simulink model "k1visetmyp"  (Simulink 8.6)
settings: Solver=ode45  StartTime=0.0  StopTime=10.0  RelTol=1e-3
libraries: cdsIPCx x50, cdsFilt x11, cdsCDI64 x6, cdsCDO64 x6, BIO_CD_DECODE_MASTER x6, BIO_CD_ENCODE_MASTER x5, CHK_DIO x5, dac x3, cdsBit2Word x2, cdsAdcx0 x1, cdsAdcx1 x1, TYPEA_MASTER x1
(part 1 of 2)
settings Model: Creator=controls  LastModifiedBy=controls
settings DataIOCC: SignalLoggingSaveFormat=Dataset
settings OptimizationCC: ExpressionDepthLimit=128
settings DebuggingCC: UnderspecifiedInitializationDetection=Simplified  MergeDetectMultiDrivingBlocksExec=error  SolverPrmCheckMsg=none  FcnCallInpInsideContextMsg=EnableAllAsError  StateNameClashWarn=none
settings GRTTargetCC: CombineOutputUpdateFcns=on  GRTInterface=off

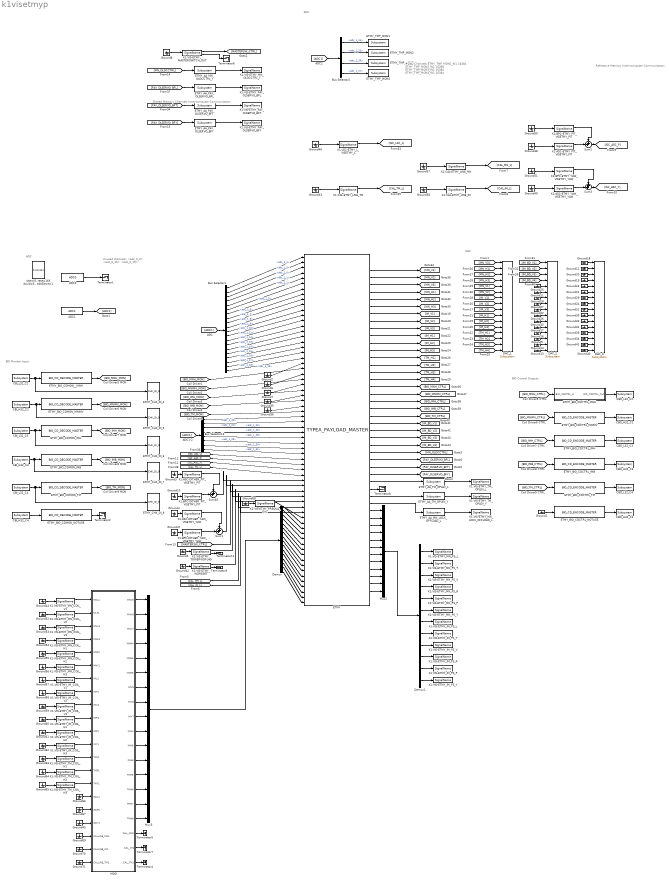
== system k1visetmyp ==
  note: BIO Monitor Input
  note: BIO Control Outputs
  note: DAC
  note: ADC
  note: Refrective Memory
      | Inner-computer Communication
  note: Unused channels:
      | <adc_0_3>
      | <adc_0_15>
      | <adc_0_19>
  note: Shared Memory Channels
      | Inner-computer Communication
  note: #DAQ Channels
      | ETMY_TMP_MON1_IN1 16384
      | ETMY_TMP_MON2_IN1 16384
      | ETMY_TMP_MON3_IN1 16384
      | ETMY_TMP_MON4_IN1 16384
  note: ADC
  ADC0 : cdsAdcx0/ADC0  Tag=cdsAdc  Description=|
      | type-GSC_16AI64SSA
      | card_num=0
      settings: AttributesFormatString=%<Description>\n%<Tag>
  ADC1 : cdsAdcx1/ADC1  Tag=cdsAdc  Description=|
      | type-GSC_16AI64SSA
      | card_num=1
      settings: AttributesFormatString=%<Description>\n%<Tag>
  Bus Selector1 : BusSelector  OutputSignals=adc_1_4,adc_1_5,adc_1_0,adc_1_1,adc_1_2,adc_1_3,adc_1_6,adc_1_7,adc_1_8,adc_1_9,adc_1_10,adc_1_11,adc_1_12,adc_1_13,adc_1_14,adc_1_15,adc_1_16,adc_1_17,adc_1_18,adc_1_19
  Bus Selector13 : BusSelector  OutputSignals=adc_1_20,adc_1_21,adc_1_22,adc_1_23,adc_1_28,adc_1_29,adc_1_30,adc_1_31
  Bus Selector2 : BusSelector  OutputSignals=adc_1_24,adc_1_25,adc_1_26,adc_1_27
  CBI_H32_C2 : cdsCDI64/Subsystem  Tag=cdsCDI64  Description=card_num=5
      settings: AttributesFormatString=%<Tag>\n%<Description>
  CBI_H32_C3 : cdsCDI64/Subsystem  Tag=cdsCDI64  Description=card_num=7
      settings: AttributesFormatString=%<Tag>\n%<Description>
  CBI_H32_C4 : cdsCDI64/Subsystem  Tag=cdsCDI64  Description=card_num=9
      settings: AttributesFormatString=%<Tag>\n%<Description>
  CBI_L32_C2 : cdsCDI64/Subsystem  Tag=cdsCDI64  Description=card_num=4
      settings: AttributesFormatString=%<Tag>\n%<Description>
  CBI_L32_C3 : cdsCDI64/Subsystem  Tag=cdsCDI64  Description=card_num=6
      settings: AttributesFormatString=%<Tag>\n%<Description>
  CBI_L32_C4 : cdsCDI64/Subsystem  Tag=cdsCDI64  Description=card_num=8
      settings: AttributesFormatString=%<Tag>\n%<Description>
  CBO_H32_C2 : cdsCDO64/Subsystem  Tag=cdsCDO64  Description=card_num=5
      settings: AttributesFormatString=%<Tag>\n%<Description>
  CBO_H32_C3 : cdsCDO64/Subsystem  Tag=cdsCDO64  Description=card_num=7
      settings: AttributesFormatString=%<Tag>\n%<Description>
  CBO_H32_C4 : cdsCDO64/Subsystem  Tag=cdsCDO64  Description=card_num=9
      settings: AttributesFormatString=%<Tag>\n%<Description>
  CBO_L32_C2 : cdsCDO64/Subsystem  Tag=cdsCDO64  Description=card_num=4
      settings: AttributesFormatString=%<Tag>\n%<Description>
  CBO_L32_C3 : cdsCDO64/Subsystem  Tag=cdsCDO64  Description=card_num=6
      settings: AttributesFormatString=%<Tag>\n%<Description>
  CBO_L32_C4 : cdsCDO64/Subsystem  Tag=cdsCDO64  Description=card_num=8
      settings: AttributesFormatString=%<Tag>\n%<Description>
  DAC_0 : dac/Subsystem  Description=|
      | type=GSC_16AO16,
      | card_num=0
      settings: AttributesFormatString=%<Description>
  DAC_1 : dac/Subsystem  Description=|
      | type=GSC_16AO16,
      | card_num=1
      settings: AttributesFormatString=%<Description>
  DAC_2 : dac/Subsystem  Description=|
      | type=GSC_16AO16,
      | card_num=2
      settings: AttributesFormatString=%<Description>
  Demux : Demux  Outputs=16
  Demux1 : Demux  Outputs=12
  ETMY : TYPEA_MASTER/TYPEA_PAYLOAD_MASTER
  ETMY_AA_MN_LOCK_OFFLOAD_L : cdsFilt/Subsystem  Tag=cdsFilt  Description=|
      | Purpose:                                                                                                                                                                                                                                  
      | Standard CDS IIR filter module.                                                                                                                                                                                                           
      |                                                                                                                                                                                                                                           
      | Operation:                                                                                                                                                                                                                                
      | Consists of 10 second order section IIR filters, plus a ramped gain stage. In FE code, also provides pre-defined test points and excitation channel inputs. The filter coefficients are defined in the LIGO system using the 'foton' tool.
      |                                                                                                                                                                                                                                           
      | Usage:                                                                                                                                                                                                                                    
      | Name the part with the desired filter module name.
      settings: AttributesFormatString=%<Tag>
  ETMY_AA_MN_OLDCCTRL_Y : cdsFilt/Subsystem  Tag=cdsFilt  Description=|
      | Purpose:                                                                                                                                                                                                                                  
      | Standard CDS IIR filter module.                                                                                                                                                                                                           
      |                                                                                                                                                                                                                                           
      | Operation:                                                                                                                                                                                                                                
      | Consists of 10 second order section IIR filters, plus a ramped gain stage. In FE code, also provides pre-defined test points and excitation channel inputs. The filter coefficients are defined in the LIGO system using the 'foton' tool.
      |                                                                                                                                                                                                                                           
      | Usage:                                                                                                                                                                                                                                    
      | Name the part with the desired filter module name.
      settings: AttributesFormatString=%<Tag>
  ETMY_AA_PAY_OLSERVO_BFL : cdsFilt/Subsystem  Tag=cdsFilt  Description=|
      | Purpose:                                                                                                                                                                                                                                  
      | Standard CDS IIR filter module.                                                                                                                                                                                                           
      |                                                                                                                                                                                                                                           
      | Operation:                                                                                                                                                                                                                                
      | Consists of 10 second order section IIR filters, plus a ramped gain stage. In FE code, also provides pre-defined test points and excitation channel inputs. The filter coefficients are defined in the LIGO system using the 'foton' tool.
      |                                                                                                                                                                                                                                           
      | Usage:                                                                                                                                                                                                                                    
      | Name the part with the desired filter module name.
      settings: AttributesFormatString=%<Tag>
  ETMY_AA_PAY_OLSERVO_BFT : cdsFilt/Subsystem  Tag=cdsFilt  Description=|
      | Purpose:                                                                                                                                                                                                                                  
      | Standard CDS IIR filter module.                                                                                                                                                                                                           
      |                                                                                                                                                                                                                                           
      | Operation:                                                                                                                                                                                                                                
      | Consists of 10 second order section IIR filters, plus a ramped gain stage. In FE code, also provides pre-defined test points and excitation channel inputs. The filter coefficients are defined in the LIGO system using the 'foton' tool.
      |                                                                                                                                                                                                                                           
      | Usage:                                                                                                                                                                                                                                    
      | Name the part with the desired filter module name.
      settings: AttributesFormatString=%<Tag>
  ETMY_AA_PAY_OLSERVO_BFY : cdsFilt/Subsystem  Tag=cdsFilt  Description=|
      | Purpose:                                                                                                                                                                                                                                  
      | Standard CDS IIR filter module.                                                                                                                                                                                                           
      |                                                                                                                                                                                                                                           
      | Operation:                                                                                                                                                                                                                                
      | Consists of 10 second order section IIR filters, plus a ramped gain stage. In FE code, also provides pre-defined test points and excitation channel inputs. The filter coefficients are defined in the LIGO system using the 'foton' tool.
      |                                                                                                                                                                                                                                           
      | Usage:                                                                                                                                                                                                                                    
      | Name the part with the desired filter module name.
      settings: AttributesFormatString=%<Tag>
  ETMY_AA_TM_OPLEV_L : cdsFilt/Subsystem  Tag=cdsFilt  Description=|
      | Purpose:                                                                                                                                                                                                                                  
      | Standard CDS IIR filter module.                                                                                                                                                                                                           
      |                                                                                                                                                                                                                                           
      | Operation:                                                                                                                                                                                                                                
      | Consists of 10 second order section IIR filters, plus a ramped gain stage. In FE code, also provides pre-defined test points and excitation channel inputs. The filter coefficients are defined in the LIGO system using the 'foton' tool.
      |                                                                                                                                                                                                                                           
      | Usage:                                                                                                                                                                                                                                    
      | Name the part with the desired filter module name.
      settings: AttributesFormatString=%<Tag>
  ETMY_AA_TM_OPLEV_Y : cdsFilt/Subsystem  Tag=cdsFilt  Description=|
      | Purpose:                                                                                                                                                                                                                                  
      | Standard CDS IIR filter module.                                                                                                                                                                                                           
      |                                                                                                                                                                                                                                           
      | Operation:                                                                                                                                                                                                                                
      | Consists of 10 second order section IIR filters, plus a ramped gain stage. In FE code, also provides pre-defined test points and excitation channel inputs. The filter coefficients are defined in the LIGO system using the 'foton' tool.
      |                                                                                                                                                                                                                                           
      | Usage:                                                                                                                                                                                                                                    
      | Name the part with the desired filter module name.
      settings: AttributesFormatString=%<Tag>
  ETMY_BIO_CDCTRL_IMB : BIO_CD_ENCODE_MASTER/BIO_CD_ENCODE_MASTER
  ETMY_BIO_CDCTRL_IMH : BIO_CD_ENCODE_MASTER/BIO_CD_ENCODE_MASTER
  ETMY_BIO_CDCTRL_MNH : Subsystem
  ETMY_BIO_CDCTRL_MNIMV : BIO_CD_ENCODE_MASTER/BIO_CD_ENCODE_MASTER
  ETMY_BIO_CDCTRL_NOTUSE : BIO_CD_ENCODE_MASTER/BIO_CD_ENCODE_MASTER
  ETMY_BIO_CDCTRL_TM : BIO_CD_ENCODE_MASTER/BIO_CD_ENCODE_MASTER
  ETMY_BIO_CDMON_IMB : BIO_CD_DECODE_MASTER/BIO_CD_DECODE_MASTER
  ETMY_BIO_CDMON_IMH : BIO_CD_DECODE_MASTER/BIO_CD_DECODE_MASTER
  ETMY_BIO_CDMON_MNIMV : BIO_CD_DECODE_MASTER/BIO_CD_DECODE_MASTER
  ETMY_BIO_CDMON_NOTUSE : BIO_CD_DECODE_MASTER/BIO_CD_DECODE_MASTER
  ETMY_BIO_CDMON_TM : BIO_CD_DECODE_MASTER/BIO_CD_DECODE_MASTER
  ETMY_BIO_CDMON__MNH : BIO_CD_DECODE_MASTER/BIO_CD_DECODE_MASTER
  ETMY_CHK_DI_{4..8} (5 alike) : CHK_DIO/CHK_DI_0
  ETMY_TMP_MON1 : cdsFilt/Subsystem  Tag=cdsFilt  Description=|
      | Purpose:                                                                                                                                                                                                                                  
      | Standard CDS IIR filter module.                                                                                                                                                                                                           
      |                                                                                                                                                                                                                                           
      | Operation:                                                                                                                                                                                                                                
      | Consists of 10 second order section IIR filters, plus a ramped gain stage. In FE code, also provides pre-defined test points and excitation channel inputs. The filter coefficients are defined in the LIGO system using the 'foton' tool.
      |                                                                                                                                                                                                                                           
      | Usage:                                                                                                                                                                                                                                    
      | Name the part with the desired filter module name.
      settings: AttributesFormatString=%<Tag>
  ETMY_TMP_MON2 : cdsFilt/Subsystem  Tag=cdsFilt  Description=|
      | Purpose:                                                                                                                                                                                                                                  
      | Standard CDS IIR filter module.                                                                                                                                                                                                           
      |                                                                                                                                                                                                                                           
      | Operation:                                                                                                                                                                                                                                
      | Consists of 10 second order section IIR filters, plus a ramped gain stage. In FE code, also provides pre-defined test points and excitation channel inputs. The filter coefficients are defined in the LIGO system using the 'foton' tool.
      |                                                                                                                                                                                                                                           
      | Usage:                                                                                                                                                                                                                                    
      | Name the part with the desired filter module name.
      settings: AttributesFormatString=%<Tag>
  ETMY_TMP_MON3 : cdsFilt/Subsystem  Tag=cdsFilt  Description=|
      | Purpose:                                                                                                                                                                                                                                  
      | Standard CDS IIR filter module.                                                                                                                                                                                                           
      |                                                                                                                                                                                                                                           
      | Operation:                                                                                                                                                                                                                                
      | Consists of 10 second order section IIR filters, plus a ramped gain stage. In FE code, also provides pre-defined test points and excitation channel inputs. The filter coefficients are defined in the LIGO system using the 'foton' tool.
      |                                                                                                                                                                                                                                           
      | Usage:                                                                                                                                                                                                                                    
      | Name the part with the desired filter module name.
      settings: AttributesFormatString=%<Tag>
  ETMY_TMP_MON4 : cdsFilt/Subsystem  Tag=cdsFilt  Description=|
      | Purpose:                                                                                                                                                                                                                                  
      | Standard CDS IIR filter module.                                                                                                                                                                                                           
      |                                                                                                                                                                                                                                           
      | Operation:                                                                                                                                                                                                                                
      | Consists of 10 second order section IIR filters, plus a ramped gain stage. In FE code, also provides pre-defined test points and excitation channel inputs. The filter coefficients are defined in the LIGO system using the 'foton' tool.
      |                                                                                                                                                                                                                                           
      | Usage:                                                                                                                                                                                                                                    
      | Name the part with the desired filter module name.
      settings: AttributesFormatString=%<Tag>
  Ground{1..71} (71 alike) : Ground
  K1:ASC-DITHER_PIT_VISETMY_PIT : cdsIPCx/SignalName  Tag=cdsIPCx_RFM  Description=card=1
      settings: AttributesFormatString=%<Description>\n%<Tag>
  K1:ASC-DITHER_YAW_VISETMY_YAW : cdsIPCx/SignalName  Tag=cdsIPCx_RFM  Description=card=1
      settings: AttributesFormatString=%<Description>\n%<Tag>
  K1:ASC-ETMY_PIT_VISETMY_PIT : cdsIPCx/SignalName  Tag=cdsIPCx_RFM  Description=card=1
      settings: AttributesFormatString=%<Description>\n%<Tag>
  K1:ASC-ETMY_YAW_VISETMY_YAW : cdsIPCx/SignalName  Tag=cdsIPCx_RFM  Description=card=1
      settings: AttributesFormatString=%<Description>\n%<Tag>
  K1:BPC-DITHER_PIT_VISETMY_PIT : cdsIPCx/SignalName  Tag=cdsIPCx_RFM  Description=card=1
      settings: AttributesFormatString=%<Description>\n%<Tag>
  K1:BPC-DITHER_YAW_VISETMY_YAW : cdsIPCx/SignalName  Tag=cdsIPCx_RFM  Description=card=1
      settings: AttributesFormatString=%<Description>\n%<Tag>
  K1:BPC-ETMY_PIT_VISETMY_PIT : cdsIPCx/SignalName  Tag=cdsIPCx_RFM  Description=card=1
      settings: AttributesFormatString=%<Description>\n%<Tag>
  K1:BPC-ETMY_YAW_VISETMY_YAW : cdsIPCx/SignalName  Tag=cdsIPCx_RFM  Description=card=1
      settings: AttributesFormatString=%<Description>\n%<Tag>
  K1:CAL-ETMY_LINE_IM : cdsIPCx/SignalName  Tag=cdsIPCx_RFM  Description=card=1
      settings: AttributesFormatString=%<Description>\n%<Tag>
  K1:CAL-ETMY_LINE_MN : cdsIPCx/SignalName  Tag=cdsIPCx_RFM  Description=card=1
      settings: AttributesFormatString=%<Description>\n%<Tag>
  K1:CAL-ETMY_LINE_TM : cdsIPCx/SignalName  Tag=cdsIPCx_RFM  Description=card=1
      settings: AttributesFormatString=%<Description>\n%<Tag>
  K1:LSC-ETMY_L_VISETMY_L : cdsIPCx/SignalName  Tag=cdsIPCx_RFM  Description=card=1
      settings: AttributesFormatString=%<Description>\n%<Tag>
  K1:VIS-ETMY_IM_COIL_H1 : cdsIPCx/SignalName  Tag=cdsIPCx_SHMEM  Description=Inter-Process Communication via Shared memory.
      settings: AttributesFormatString=%<Tag>
  K1:VIS-ETMY_IM_COIL_H2 : cdsIPCx/SignalName  Tag=cdsIPCx_SHMEM  Description=Inter-Process Communication via Shared memory.
      settings: AttributesFormatString=%<Tag>
  K1:VIS-ETMY_IM_COIL_H3 : cdsIPCx/SignalName  Tag=cdsIPCx_SHMEM  Description=Inter-Process Communication via Shared memory.
      settings: AttributesFormatString=%<Tag>
  K1:VIS-ETMY_IM_COIL_V1 : cdsIPCx/SignalName  Tag=cdsIPCx_SHMEM  Description=Inter-Process Communication via Shared memory.
      settings: AttributesFormatString=%<Tag>
  K1:VIS-ETMY_IM_COIL_V2 : cdsIPCx/SignalName  Tag=cdsIPCx_SHMEM  Description=Inter-Process Communication via Shared memory.
      settings: AttributesFormatString=%<Tag>
  K1:VIS-ETMY_IM_COIL_V3 : cdsIPCx/SignalName  Tag=cdsIPCx_SHMEM  Description=Inter-Process Communication via Shared memory.
      settings: AttributesFormatString=%<Tag>
  K1:VIS-ETMY_MN_COIL_H1 : cdsIPCx/SignalName  Tag=cdsIPCx_SHMEM  Description=Inter-Process Communication via Shared memory.
      settings: AttributesFormatString=%<Tag>
  K1:VIS-ETMY_MN_COIL_H2 : cdsIPCx/SignalName  Tag=cdsIPCx_SHMEM  Description=Inter-Process Communication via Shared memory.
      settings: AttributesFormatString=%<Tag>
  K1:VIS-ETMY_MN_COIL_H3 : cdsIPCx/SignalName  Tag=cdsIPCx_SHMEM  Description=Inter-Process Communication via Shared memory.
      settings: AttributesFormatString=%<Tag>
  K1:VIS-ETMY_MN_COIL_V1 : cdsIPCx/SignalName  Tag=cdsIPCx_SHMEM  Description=Inter-Process Communication via Shared memory.
      settings: AttributesFormatString=%<Tag>
  K1:VIS-ETMY_MN_COIL_V2 : cdsIPCx/SignalName  Tag=cdsIPCx_SHMEM  Description=Inter-Process Communication via Shared memory.
      settings: AttributesFormatString=%<Tag>
  K1:VIS-ETMY_MN_COIL_V3 : cdsIPCx/SignalName  Tag=cdsIPCx_SHMEM  Description=Inter-Process Communication via Shared memory.
      settings: AttributesFormatString=%<Tag>
  K1:VIS-ETMY_TM_COIL_H1 : cdsIPCx/SignalName  Tag=cdsIPCx_SHMEM  Description=Inter-Process Communication via Shared memory.
      settings: AttributesFormatString=%<Tag>
  K1:VIS-ETMY_TM_COIL_H2 : cdsIPCx/SignalName  Tag=cdsIPCx_SHMEM  Description=Inter-Process Communication via Shared memory.
      settings: AttributesFormatString=%<Tag>
  K1:VIS-ETMY_TM_COIL_H3 : cdsIPCx/SignalName  Tag=cdsIPCx_SHMEM  Description=Inter-Process Communication via Shared memory.
      settings: AttributesFormatString=%<Tag>
  K1:VIS-ETMY_IM_PS_L : cdsIPCx/SignalName  Tag=cdsIPCx_SHMEM  Description=Inter-Process Communication via Shared memory.
      settings: AttributesFormatString=%<Tag>
  K1:VIS-ETMY_IM_PS_P : cdsIPCx/SignalName  Tag=cdsIPCx_SHMEM  Description=Inter-Process Communication via Shared memory.
      settings: AttributesFormatString=%<Tag>
  K1:VIS-ETMY_IM_PS_R : cdsIPCx/SignalName  Tag=cdsIPCx_SHMEM  Description=Inter-Process Communication via Shared memory.
      settings: AttributesFormatString=%<Tag>
  K1:VIS-ETMY_IM_PS_T : cdsIPCx/SignalName  Tag=cdsIPCx_SHMEM  Description=Inter-Process Communication via Shared memory.
      settings: AttributesFormatString=%<Tag>
  K1:VIS-ETMY_IM_PS_V : cdsIPCx/SignalName  Tag=cdsIPCx_SHMEM  Description=Inter-Process Communication via Shared memory.
      settings: AttributesFormatString=%<Tag>
  K1:VIS-ETMY_IM_PS_Y : cdsIPCx/SignalName  Tag=cdsIPCx_SHMEM  Description=Inter-Process Communication via Shared memory.
      settings: AttributesFormatString=%<Tag>
  K1:VIS-ETMY_MASTERSWITCH_OUT : cdsIPCx/SignalName  Tag=cdsIPCx_SHMEM  Description=Inter-Process Communication via Shared memory.
      settings: AttributesFormatString=%<Tag>
  K1:VIS-ETMY_MN_LOCK_OFFLOAD_L : cdsIPCx/SignalName  Tag=cdsIPCx_SHMEM  Description=Inter-Process Communication via Shared memory.
      settings: AttributesFormatString=%<Tag>
  K1:VIS-ETMY_MN_OLDCCTRL_Y : cdsIPCx/SignalName  Tag=cdsIPCx_SHMEM  Description=Inter-Process Communication via Shared memory.
      settings: AttributesFormatString=%<Tag>
  K1:VIS-ETMY_MN_PS_L : cdsIPCx/SignalName  Tag=cdsIPCx_SHMEM  Description=Inter-Process Communication via Shared memory.
      settings: AttributesFormatString=%<Tag>
  K1:VIS-ETMY_MN_PS_P : cdsIPCx/SignalName  Tag=cdsIPCx_SHMEM  Description=Inter-Process Communication via Shared memory.
      settings: AttributesFormatString=%<Tag>
  K1:VIS-ETMY_MN_PS_R : cdsIPCx/SignalName  Tag=cdsIPCx_SHMEM  Description=Inter-Process Communication via Shared memory.
      settings: AttributesFormatString=%<Tag>
  K1:VIS-ETMY_MN_PS_T : cdsIPCx/SignalName  Tag=cdsIPCx_SHMEM  Description=Inter-Process Communication via Shared memory.
      settings: AttributesFormatString=%<Tag>
  K1:VIS-ETMY_MN_PS_V : cdsIPCx/SignalName  Tag=cdsIPCx_SHMEM  Description=Inter-Process Communication via Shared memory.
      settings: AttributesFormatString=%<Tag>
  K1:VIS-ETMY_MN_PS_Y : cdsIPCx/SignalName  Tag=cdsIPCx_SHMEM  Description=Inter-Process Communication via Shared memory.
      settings: AttributesFormatString=%<Tag>
  K1:VIS-ETMY_PAY_OLSERVO_BFL : cdsIPCx/SignalName  Tag=cdsIPCx_SHMEM  Description=Inter-Process Communication via Shared memory.
      settings: AttributesFormatString=%<Tag>
  K1:VIS-ETMY_PAY_OLSERVO_BFT : cdsIPCx/SignalName  Tag=cdsIPCx_SHMEM  Description=Inter-Process Communication via Shared memory.
      settings: AttributesFormatString=%<Tag>
  K1:VIS-ETMY_PAY_OLSERVO_BFY : cdsIPCx/SignalName  Tag=cdsIPCx_SHMEM  Description=Inter-Process Communication via Shared memory.
      settings: AttributesFormatString=%<Tag>
  K1:VIS-ETMY_PREQUA_EXC : cdsIPCx/SignalName  Tag=cdsIPCx_SHMEM  Description=Inter-Process Communication via Shared memory.
      settings: AttributesFormatString=%<Tag>
  K1:VIS-ETMY_TM_OPLEV_L : cdsIPCx/SignalName  Tag=cdsIPCx_SHMEM  Description=Inter-Process Communication via Shared memory.
      settings: AttributesFormatString=%<Tag>
  K1:VIS-ETMY_TM_OPLEV_Y : cdsIPCx/SignalName  Tag=cdsIPCx_SHMEM  Description=Inter-Process Communication via Shared memory.
      settings: AttributesFormatString=%<Tag>
  K1:VIS-ETMY_TOWERWDFLAG : cdsIPCx/SignalName  Tag=cdsIPCx_SHMEM  Description=Inter-Process Communication via Shared memory.
      settings: AttributesFormatString=%<Tag>
  K1:VIS-ETMY_WDRESET : cdsIPCx/SignalName  Tag=cdsIPCx_SHMEM  Description=Inter-Process Communication via Shared memory.
      settings: AttributesFormatString=%<Tag>
  MOD : Subsystem  Tag=top_names
  Mux2 : Mux  Inputs=12
  Mux3 : Mux  Inputs=16
  Sum{1..3,45} (4 alike) : Sum  Inputs=++|
  Terminator{1..8,12} (9 alike) : Terminator
  site=K1 rate=16K dcuid=64 host=k1ey1 specific_cpu=3 adcSlave=1 : cdsParameters/Subsystem  Tag=cdsParameters  Description=|
      | Purpose:                                                                                                                                                                                                                                
      | Provide system parameters to the FE code generator to properly configure the generated EPICS names, rep rate of the FE controller, and the Data Acquisition node ID for proper storage of data from this FE controller.                 
      |                                                                                                                                                                                                                                         
      | Useage:                                                                                                                                                                                                                                 
      | The part NAME field is used to identify the FE parameters. It must be of the form:                                                                                                                                                      
      | site=                                                                                                                                                                                                                                   
      | rate=                                                                                                                                                                                                                                   
      | dcuid=                                                                                                                                                                                                                                  
      |                                                                                                                                                                                                                                         
      | Where:                                                                                                                                                                                                                                  
      | site= argument may be H1, H2, L1, M1, G1, either as a single argument or multiple, for example site=H1,H2. These are the only names allowed. These will become the first two characters of all EPICS and signal names (for example G1:).
      |                                                                                                                                                                                                                                         
      | rate= may be 2K, 16K, 32K, or 64K                                                                                                                                                                                                       
      |                                                                                                                                                                                                                                         
      | dcuid= is site specific ie it must be unique at each site.
      settings: AttributesFormatString=%<Tag>
  wires:
  ADC1/1 -> [ADC1]
  ETMY/1 -> [MN_V1]
  ETMY/2 -> [MN_V2]
  ETMY/3 -> [MN_V3]
  ETMY/4 -> [MN_H1]
  ETMY/6 -> [MN_H3]
  ETMY/7 -> [IM_V1]
  ETMY/8 -> [IM_V2]
  ETMY/9 -> [IM_V3]
  ETMY/11 -> [IM_H2]
  ETMY/12 -> [IM_H3]
  ETMY/13 -> [TM_H1]
  ETMY/14 -> [TM_H2]
  ETMY/16 -> [TM_H4]
  ETMY/17 -> [BIO_MNH_CTRL]
  ETMY/19 -> [BIO_IMH_CTRL]
  ETMY/18 -> [BIO_MNIMV_CTRL]
  ETMY/20 -> [BIO_IMB_CTRL]
  ETMY/21 -> [BIO_TM_CTRL]
  [ADC1] -> Bus Selector13/1
  [MN_V3] -> DAC_1/1
  [MN_H1] -> DAC_1/2
  [MN_H2] -> DAC_1/3
  [MN_H3] -> DAC_1/4
  [MN_V1] -> DAC_1/5
  [MN_V2] -> DAC_1/6
  [IM_V1] -> DAC_1/7
  [IM_V2] -> DAC_1/8
  [IM_V3] -> DAC_1/9
  [IM_H1] -> DAC_1/10
  [TM_H1] -> DAC_1/13
  [TM_H4] -> DAC_1/16
  [TM_H3] -> DAC_1/15
  [TM_H2] -> DAC_1/14
  [IM_H2] -> DAC_1/11
  [IM_H3] -> DAC_1/12
  [BIO_MNH_CTRL] -> ETMY_BIO_CDCTRL_MNH/1(BIO_CDCTRL_In)
  ETMY_BIO_CDCTRL_MNH/1(DIO_CDCTRL_Out) -> CBO_L32_C2/1
  [BIO_MNIMV_CTRL] -> ETMY_BIO_CDCTRL_MNIMV/1
  ETMY_BIO_CDCTRL_MNIMV/1 -> CBO_H32_C2/1
  [BIO_IMH_CTRL] -> ETMY_BIO_CDCTRL_IMH/1
  ETMY_BIO_CDCTRL_IMH/1 -> CBO_L32_C3/1
  [BIO_IMB_CTRL] -> ETMY_BIO_CDCTRL_IMB/1
  ETMY_BIO_CDCTRL_IMB/1 -> CBO_H32_C3/1
  [BIO_TM_CTRL] -> ETMY_BIO_CDCTRL_TM/1
  ETMY_BIO_CDCTRL_TM/1 -> CBO_L32_C4/1
  Ground1/1 -> ETMY_BIO_CDCTRL_NOTUSE/1
  ETMY_BIO_CDCTRL_NOTUSE/1 -> CBO_H32_C4/1
  CBI_L32_C2/1 -> ETMY_CHK_DI_4/1, ETMY_BIO_CDMON__MNH/1
  ETMY_BIO_CDMON__MNH/1 -> [BIO_MNH_MON]
  CBI_H32_C2/1 -> ETMY_CHK_DI_5/1, ETMY_BIO_CDMON_MNIMV/1
  ETMY_BIO_CDMON_MNIMV/1 -> [BIO_MNIMV_MON]
  CBI_L32_C3/1 -> ETMY_CHK_DI_6/1, ETMY_BIO_CDMON_IMH/1
  ETMY_BIO_CDMON_IMH/1 -> [BIO_IMH_MON]
  ETMY_BIO_CDMON_IMB/1 -> [BIO_IMB_MON]
  CBI_L32_C4/1 -> ETMY_CHK_DI_8/1, ETMY_BIO_CDMON_TM/1
  ETMY_BIO_CDMON_TM/1 -> [BIO_TM_MON]
  CBI_H32_C4/1 -> ETMY_BIO_CDMON_NOTUSE/1
  ETMY_BIO_CDMON_NOTUSE/1 -> Terminator2/1
  [IM_BD_V1] -> DAC_2/1
  [IM_BD_V2] -> DAC_2/2
  [IM_BD_V3] -> DAC_2/3
  [IM_BD_V4] -> DAC_2/4
  Ground25/1 -> DAC_2/5
  Ground11/1 -> DAC_2/6
  Ground28/1 -> DAC_2/7
  Ground27/1 -> DAC_2/8
  Ground22/1 -> DAC_2/9
  Ground26/1 -> DAC_2/10
  Ground15/1 -> DAC_2/11
  Ground17/1 -> DAC_2/12
  Ground16/1 -> DAC_2/13
  Ground9/1 -> DAC_2/14
  Ground14/1 -> DAC_2/15
  Ground13/1 -> DAC_2/16
  ETMY/22 -> [IM_BD_V1]
  ETMY/23 -> [IM_BD_V2]
  ETMY/24 -> [IM_BD_V3]
  ETMY/25 -> [IM_BD_V4]
  CBI_H32_C3/1 -> ETMY_CHK_DI_7/1, ETMY_BIO_CDMON_IMB/1
  ETMY/5 -> [MN_H2]
  ETMY/10 -> [IM_H1]
  ETMY/15 -> [TM_H3]
  [ADC1] -> Bus Selector1/1
  Bus Selector1/1 -> ETMY/1  "<adc_1_4>"
  Bus Selector1/2 -> ETMY/2  "<adc_1_5>"
  Bus Selector1/3 -> ETMY/3  "<adc_1_0>"
  Bus Selector1/4 -> ETMY/4  "<adc_1_1>"
  Bus Selector1/5 -> ETMY/5  "<adc_1_2>"
  Bus Selector1/6 -> ETMY/6  "<adc_1_3>"
  Bus Selector1/7 -> ETMY/7  "<adc_1_6>"
  Bus Selector1/8 -> ETMY/8  "<adc_1_7>"
  Bus Selector1/9 -> ETMY/9  "<adc_1_8>"
  Bus Selector1/10 -> ETMY/10  "<adc_1_9>"
  Bus Selector1/11 -> ETMY/11  "<adc_1_10>"
  Bus Selector1/12 -> ETMY/12  "<adc_1_11>"
  Bus Selector1/13 -> ETMY/13  "<adc_1_12>"
  Bus Selector1/14 -> ETMY/14  "<adc_1_13>"
  Bus Selector1/15 -> ETMY/15  "<adc_1_14>"
  Bus Selector1/16 -> ETMY/16  "<adc_1_15>"
  Bus Selector1/17 -> ETMY/17  "<adc_1_16>"
  Bus Selector1/18 -> ETMY/18  "<adc_1_17>"
  Bus Selector1/19 -> ETMY/19  "<adc_1_18>"
  Bus Selector1/20 -> ETMY/20  "<adc_1_19>"
  [BIO_MNH_MON] -> ETMY/22
  [BIO_MNIMV_MON] -> ETMY/24
  [BIO_IMH_MON] -> ETMY/26
  [BIO_IMB_MON] -> ETMY/28
  [BIO_TM_MON] -> ETMY/30
  Bus Selector13/2 -> ETMY/32  "<adc_1_21>"
  Bus Selector13/3 -> ETMY/33  "<adc_1_22>"
  Bus Selector13/4 -> ETMY/34  "<adc_1_23>"
  Bus Selector13/5 -> ETMY/35  "<adc_1_28>"
  Bus Selector13/6 -> ETMY/36  "<adc_1_29>"
  Bus Selector13/7 -> ETMY/37  "<adc_1_30>"
  Bus Selector13/8 -> ETMY/38  "<adc_1_31>"
  Bus Selector13/1 -> ETMY/31  "<adc_1_20>"
  [ISC_ASC_P] -> ETMY/40
  [ISC_ASC_Y] -> ETMY/41
  K1:VIS-ETMY_TOWERWDFLAG/2 -> Terminator12/1
  Ground5/1 -> K1:VIS-ETMY_TOWERWDFLAG/1
  ADC0/1 -> Terminator1/1
  Ground18/1 -> DAC_0/1
  Ground12/1 -> DAC_0/2
  Ground19/1 -> DAC_0/4
  Ground20/1 -> DAC_0/3
  Ground29/1 -> DAC_0/7
  Ground23/1 -> DAC_0/5
  Ground21/1 -> DAC_0/6
  Ground24/1 -> DAC_0/8
  Ground31/1 -> DAC_0/9
  Ground30/1 -> DAC_0/10
  Ground33/1 -> DAC_0/11
  Ground32/1 -> DAC_0/12
  Ground39/1 -> DAC_0/13
  Ground34/1 -> DAC_0/14
  Ground41/1 -> DAC_0/15
  Ground40/1 -> DAC_0/16
  K1:VIS-ETMY_WDRESET/2 -> Terminator3/1
  Ground42/1 -> K1:VIS-ETMY_WDRESET/1
  Ground46/1 -> K1:LSC-ETMY_L_VISETMY_L/1
  K1:LSC-ETMY_L_VISETMY_L/1 -> [ISC_LSC_L]
  K1:CAL-ETMY_LINE_TM/1 -> [CAL_TM_L]
  Ground43/1 -> K1:CAL-ETMY_LINE_TM/1
  [ISC_LSC_L] -> ETMY/39
  Ground2/1 -> ETMY/21
  Ground6/1 -> ETMY/23
  Ground7/1 -> ETMY/25
  Ground35/1 -> ETMY/27
  Ground36/1 -> ETMY/29
  K1:CAL-ETMY_LINE_MN/1 -> [CAL_MN_L]
  Ground37/1 -> K1:CAL-ETMY_LINE_MN/1
  K1:CAL-ETMY_LINE_IM/1 -> [CAL_IM_L]
  Ground38/1 -> K1:CAL-ETMY_LINE_IM/1
  K1:ASC-ETMY_PIT_VISETMY_PIT/1 -> Sum2/2
  K1:ASC-ETMY_YAW_VISETMY_YAW/1 -> Sum3/2
  Ground48/1 -> K1:ASC-ETMY_PIT_VISETMY_PIT/1
  Ground49/1 -> K1:ASC-ETMY_YAW_VISETMY_YAW/1
  Ground3/1 -> K1:ASC-DITHER_PIT_VISETMY_PIT/1
  Ground4/1 -> K1:ASC-DITHER_YAW_VISETMY_YAW/1
  ETMY_AA_MN_OLDCCTRL_Y/1 -> K1:VIS-ETMY_MN_OLDCCTRL_Y/1
  ETMY_AA_PAY_OLSERVO_BFY/1 -> K1:VIS-ETMY_PAY_OLSERVO_BFY/1
  ETMY_AA_PAY_OLSERVO_BFT/1 -> K1:VIS-ETMY_PAY_OLSERVO_BFT/1
  ETMY_AA_PAY_OLSERVO_BFL/1 -> K1:VIS-ETMY_PAY_OLSERVO_BFL/1
  [PAY_OLSERVO_BFY] -> ETMY_AA_PAY_OLSERVO_BFY/1
  [PAY_OLSERVO_BFT] -> ETMY_AA_PAY_OLSERVO_BFT/1
  [PAY_OLSERVO_BFL] -> ETMY_AA_PAY_OLSERVO_BFL/1
  [MN_OLDCCTRL] -> ETMY_AA_MN_OLDCCTRL_Y/1
  ETMY_AA_TM_OPLEV_L/1 -> K1:VIS-ETMY_TM_OPLEV_L/1
  ETMY_AA_TM_OPLEV_Y/1 -> K1:VIS-ETMY_TM_OPLEV_Y/1
  [ADC1] -> Bus Selector2/1
  Bus Selector2/1 -> ETMY_TMP_MON1/1  "<adc_1_24>"
  Bus Selector2/2 -> ETMY_TMP_MON2/1  "<adc_1_25>"
  Bus Selector2/4 -> ETMY_TMP_MON4/1  "<adc_1_27>"
  Bus Selector2/3 -> ETMY_TMP_MON3/1  "<adc_1_26>"
  ETMY/29 -> [PAY_OLSERVO_BFY]
  ETMY/26 -> [MN_OLDCCTRL]
  ETMY/27 -> [PAY_OLSERVO_BFL]
  ETMY/28 -> [PAY_OLSERVO_BFT]
  ETMY/30 -> ETMY_AA_TM_OPLEV_L/1
  ETMY/31 -> Terminator8/1
  ETMY/32 -> ETMY_AA_TM_OPLEV_Y/1
  K1:VIS-ETMY_MASTERSWITCH_OUT/1 -> [MASTERSW_CTRL]
  K1:VIS-ETMY_MASTERSWITCH_OUT/2 -> Terminator6/1
  Ground8/1 -> K1:VIS-ETMY_MASTERSWITCH_OUT/1
  [CAL_IM_L] -> ETMY/49
  ETMY/33 -> ETMY_AA_MN_LOCK_OFFLOAD_L/1
  ETMY_AA_MN_LOCK_OFFLOAD_L/1 -> K1:VIS-ETMY_MN_LOCK_OFFLOAD_L/1
  [CAL_TM_L] -> ETMY/42
  K1:ASC-DITHER_PIT_VISETMY_PIT/1 -> Sum45/1
  [MASTERSW_CTRL] -> ETMY/45
  K1:VIS-ETMY_TOWERWDFLAG/1 -> ETMY/46
  K1:VIS-ETMY_WDRESET/1 -> ETMY/47
  [CAL_MN_L] -> ETMY/48
  Ground10/1 -> K1:BPC-DITHER_PIT_VISETMY_PIT/1
  Ground47/1 -> K1:BPC-DITHER_YAW_VISETMY_YAW/1
  K1:BPC-DITHER_PIT_VISETMY_PIT/1 -> Sum45/2
  K1:BPC-DITHER_YAW_VISETMY_YAW/1 -> Sum1/2
  Sum45/1 -> ETMY/43
  K1:ASC-DITHER_YAW_VISETMY_YAW/1 -> Sum1/1
  Sum1/1 -> ETMY/44
  K1:BPC-ETMY_PIT_VISETMY_PIT/1 -> Sum2/1
  K1:BPC-ETMY_YAW_VISETMY_YAW/1 -> Sum3/1
  Ground50/1 -> K1:BPC-ETMY_PIT_VISETMY_PIT/1
  Ground51/1 -> K1:BPC-ETMY_YAW_VISETMY_YAW/1
  Sum3/1 -> [ISC_ASC_Y]
  Sum2/1 -> [ISC_ASC_P]
  Mux3/1 -> Demux/1
  Demux/1 -> ETMY/51
  Demux/2 -> ETMY/52
  Demux/3 -> ETMY/53
  Demux/4 -> ETMY/54
  Demux/5 -> ETMY/55
  Demux/6 -> ETMY/56
  Demux/7 -> ETMY/57
  Demux/8 -> ETMY/58
  Demux/9 -> ETMY/59
  Demux/10 -> ETMY/60
  Demux/11 -> ETMY/61
  Demux/12 -> ETMY/62
  Demux/13 -> ETMY/63
  Demux/14 -> ETMY/64
  Demux/15 -> ETMY/65
  Demux/16 -> ETMY/66
  Ground68/1 -> K1:VIS-ETMY_PREQUA_EXC/1
  K1:VIS-ETMY_PREQUA_EXC/1 -> ETMY/50
  Demux1/1 -> K1:VIS-ETMY_MN_PS_L/1
  Demux1/2 -> K1:VIS-ETMY_MN_PS_T/1
  Demux1/3 -> K1:VIS-ETMY_MN_PS_V/1
  Demux1/4 -> K1:VIS-ETMY_MN_PS_R/1
  Demux1/5 -> K1:VIS-ETMY_MN_PS_P/1
  Demux1/6 -> K1:VIS-ETMY_MN_PS_Y/1
  Demux1/7 -> K1:VIS-ETMY_IM_PS_L/1
  Demux1/8 -> K1:VIS-ETMY_IM_PS_T/1
  Demux1/9 -> K1:VIS-ETMY_IM_PS_V/1
  Demux1/10 -> K1:VIS-ETMY_IM_PS_R/1
  Demux1/11 -> K1:VIS-ETMY_IM_PS_P/1
  Demux1/12 -> K1:VIS-ETMY_IM_PS_Y/1
  Mux2/1 -> Demux1/1
  ETMY/34 -> Mux2/1
  ETMY/35 -> Mux2/2
  ETMY/36 -> Mux2/3
  ETMY/37 -> Mux2/4
  ETMY/38 -> Mux2/5
  ETMY/39 -> Mux2/6
  ETMY/40 -> Mux2/7
  ETMY/41 -> Mux2/8
  ETMY/42 -> Mux2/9
  ETMY/43 -> Mux2/10
  ETMY/44 -> Mux2/11
  ETMY/45 -> Mux2/12
  MOD/1(MNV5) -> Mux3/1
  MOD/2(MNV6) -> Mux3/2
  MOD/3(MNV7) -> Mux3/3
  MOD/4(MNH4) -> Mux3/4
  MOD/5(MNH5) -> Mux3/5
  MOD/6(MNH6) -> Mux3/6
  MOD/7(IMV5) -> Mux3/7
  MOD/8(IMV6) -> Mux3/8
  MOD/9(IMV7) -> Mux3/9
  MOD/10(IMH4) -> Mux3/10
  MOD/11(IMH5) -> Mux3/11
  MOD/12(IMH6) -> Mux3/12
  MOD/13(TMH5) -> Mux3/13
  MOD/14(TMH6) -> Mux3/14
  MOD/15(TMH7) -> Mux3/15
  MOD/16(TMH8) -> Mux3/16
  Ground44/1 -> K1:VIS-ETMY_MN_COIL_V1/1
  Ground52/1 -> K1:VIS-ETMY_MN_COIL_V2/1
  Ground53/1 -> K1:VIS-ETMY_MN_COIL_V3/1
  Ground54/1 -> K1:VIS-ETMY_MN_COIL_H1/1
  Ground55/1 -> K1:VIS-ETMY_MN_COIL_H2/1
  Ground56/1 -> K1:VIS-ETMY_MN_COIL_H3/1
  Ground57/1 -> K1:VIS-ETMY_IM_COIL_V1/1
  Ground58/1 -> K1:VIS-ETMY_IM_COIL_V2/1
  Ground59/1 -> K1:VIS-ETMY_IM_COIL_V3/1
  Ground60/1 -> K1:VIS-ETMY_IM_COIL_H1/1
  Ground61/1 -> K1:VIS-ETMY_IM_COIL_H2/1
  Ground62/1 -> K1:VIS-ETMY_IM_COIL_H3/1
  Ground63/1 -> K1:VIS-ETMY_TM_COIL_H1/1
  Ground64/1 -> K1:VIS-ETMY_TM_COIL_H2/1
  Ground65/1 -> K1:VIS-ETMY_TM_COIL_H3/1
  K1:VIS-ETMY_MN_COIL_V1/1 -> MOD/1(MNL1)
  K1:VIS-ETMY_MN_COIL_V2/1 -> MOD/2(MLT1)
  K1:VIS-ETMY_MN_COIL_V3/1 -> MOD/3(MNV4)
  K1:VIS-ETMY_MN_COIL_H1/1 -> MOD/4(MNR1)
  K1:VIS-ETMY_MN_COIL_H2/1 -> MOD/5(MNP1)
  K1:VIS-ETMY_MN_COIL_H3/1 -> MOD/6(MNY1)
  K1:VIS-ETMY_IM_COIL_V1/1 -> MOD/7(IML1)
  K1:VIS-ETMY_IM_COIL_V2/1 -> MOD/8(IMT1)
  K1:VIS-ETMY_IM_COIL_V3/1 -> MOD/9(IMV4)
  K1:VIS-ETMY_IM_COIL_H1/1 -> MOD/10(IMR1)
  K1:VIS-ETMY_IM_COIL_H2/1 -> MOD/11(IMP1)
  K1:VIS-ETMY_IM_COIL_H3/1 -> MOD/12(IMY1)
  K1:VIS-ETMY_TM_COIL_H1/1 -> MOD/13(TML1)
  K1:VIS-ETMY_TM_COIL_H2/1 -> MOD/14(TMP1)
  K1:VIS-ETMY_TM_COIL_H3/1 -> MOD/15(TMY1)
  Ground67/1 -> MOD/17(ISCP1)
  Ground45/1 -> MOD/18(ISCY1)
  Ground66/1 -> MOD/16(ISCL1)
  Ground69/1 -> MOD/19(CALLINE_MN1)
  Ground70/1 -> MOD/20(CALLINE_IM1)
  Ground71/1 -> MOD/21(CALLINE_TM1)
  MOD/17(CAL_MN1) -> Terminator5/1
  MOD/18(CAL_IM1) -> Terminator7/1
  MOD/19(CAL_TM1) -> Terminator4/1
